simulink model "ARCH_AT6b_artificial"  (R2019b)
settings: Solver=FixedStepAuto  StartTime=0.0  StopTime=10.0  FixedStep=fixedStepSize  RelTol=1e-3
undefined symbols (not defined in the file): ARCH_AT6b_rpmEndTime, ARCH_AT6b_rpmStartTime, ARCH_AT6b_rpmThreshold, ARCH_AT6b_speedEndTime, ARCH_AT6b_speedStartTime, ARCH_AT6b_speedThreshold, artificial_ARCH_AT6_constant
settings Model: Creator=JEDDELAN  LastModifiedBy=JEDDELAN
settings DataIOCC: SaveOutput=off  SaveTime=off  ReturnWorkspaceOutputs=off
settings DebuggingCC: ArithmeticOperatorsInVariantConditions=warning
settings SFSimCC: SimUseLocalCustomCode=off  CustomCodeUndefinedFunction=UseInterfaceOnly
settings RTWCC: RTWUseLocalCustomCode=off
settings GRTTargetCC: CombineOutputUpdateFcns=off  MatFileLogging=off

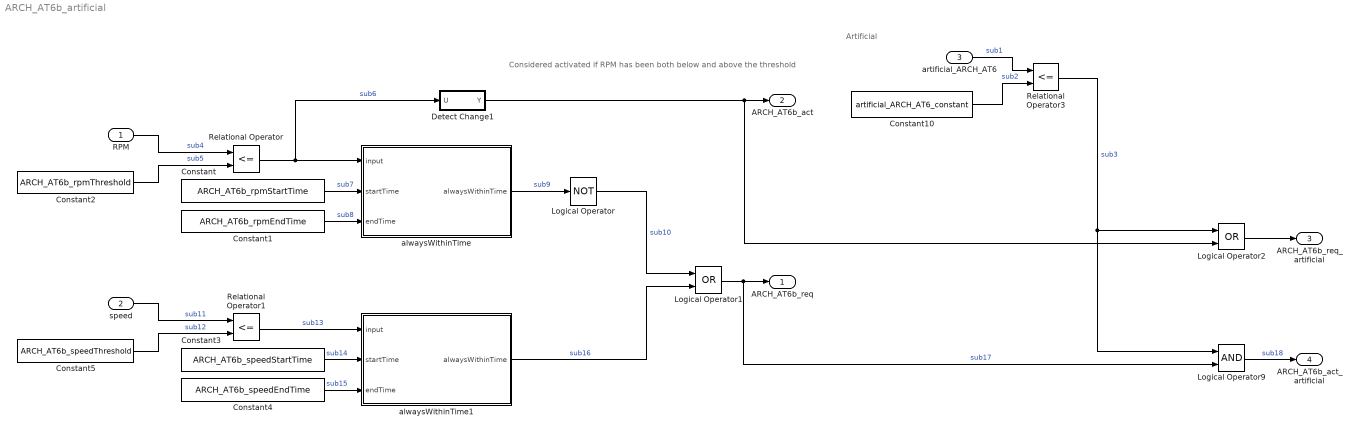
== system ARCH_AT6b_artificial ==
  note: Considered activated if RPM has been both below and above the threshold
  note: Artificial
  RPM : Inport
  speed : Inport  Port=2
  artificial_ARCH_AT6 : Inport  Port=3
  Constant : Constant  Value=ARCH_AT6b_rpmStartTime
  Constant1 : Constant  Value=ARCH_AT6b_rpmEndTime
  Constant10 : Constant  Value=artificial_ARCH_AT6_constant
  Constant2 : Constant  Value=ARCH_AT6b_rpmThreshold
  Constant3 : Constant  Value=ARCH_AT6b_speedStartTime
  Constant4 : Constant  Value=ARCH_AT6b_speedEndTime
  Constant5 : Constant  Value=ARCH_AT6b_speedThreshold
  Detect Change1 : Subsystem  mask(Detect Change){vinit=0, InputProcessing=Elements as channels (sample based), OutDataTypeStr=boolean}
      mask prompts: vinit "Simulink:masks:InitialCondition_MP"; InputProcessing "Simulink:masks:InputProcessing_MP"; OutDataTypeStr "Simulink:masks:OutputDataType_MP"
      mask help: Simulink:masks:DetectChange_MD
      mask init:
      | initDetectBlocks();
      mask TypeOptions InputProcessing: Simulink:masks:ColumnsAsChannelsFrameBased | Simulink:masks:ElementsAsChannelsSampleBased
      mask TypeOptions OutDataTypeStr: Simulink:masks:uint8 | Simulink:masks:boolean
      mask Display: fprintf('U ~= U/z')
  Logical Operator : Logic  Operator=NOT  AllPortsSameDT=off  OutDataTypeStr=boolean
  Logical Operator1 : Logic  Operator=OR  AllPortsSameDT=off  OutDataTypeStr=boolean
  Logical Operator2 : Logic  Operator=OR  AllPortsSameDT=off  OutDataTypeStr=boolean
  Logical Operator9 : Logic  AllPortsSameDT=off  OutDataTypeStr=boolean
  Relational Operator : RelationalOperator  Operator=<=  OutDataTypeStr=boolean  RndMeth=Simplest
  Relational Operator1 : RelationalOperator  Operator=<=  OutDataTypeStr=boolean  RndMeth=Simplest
  Relational Operator3 : RelationalOperator  Operator=<=  OutDataTypeStr=boolean  RndMeth=Simplest
  alwaysWithinTime : Subsystem
      settings: CopyFcn=set_param(gcbh,'LinkStatus','none');
  alwaysWithinTime1 : Subsystem
      settings: CopyFcn=set_param(gcbh,'LinkStatus','none');
  ARCH_AT6b_req : Outport  OutDataTypeStr=boolean  PortDimensions=1  VectorParamsAs1DForOutWhenUnconnected=off
  ARCH_AT6b_act : Outport  Port=2  OutDataTypeStr=boolean  PortDimensions=1  VectorParamsAs1DForOutWhenUnconnected=off
  ARCH_AT6b_req_artificial : Outport  Port=3  OutDataTypeStr=boolean  PortDimensions=1  VectorParamsAs1DForOutWhenUnconnected=off
  ARCH_AT6b_act_artificial : Outport  Port=4  OutDataTypeStr=boolean  PortDimensions=1  VectorParamsAs1DForOutWhenUnconnected=off
  wires:
  Constant1/1 -> alwaysWithinTime/3(endTime)  "sub8"
  Constant/1 -> alwaysWithinTime/2(startTime)  "sub7"
  Relational Operator/1 -> Detect Change1/1(U), alwaysWithinTime/1(input)  "sub6"
  alwaysWithinTime/1(alwaysWithinTime) -> Logical Operator/1  "sub9"
  RPM/1 -> Relational Operator/1  "sub4"
  Constant2/1 -> Relational Operator/2  "sub5"
  speed/1 -> Relational Operator1/1  "sub11"
  Relational Operator1/1 -> alwaysWithinTime1/1(input)  "sub13"
  alwaysWithinTime1/1(alwaysWithinTime) -> Logical Operator1/2  "sub16"
  Constant4/1 -> alwaysWithinTime1/3(endTime)  "sub15"
  Constant3/1 -> alwaysWithinTime1/2(startTime)  "sub14"
  Constant5/1 -> Relational Operator1/2  "sub12"
  Logical Operator/1 -> Logical Operator1/1  "sub10"
  Constant10/1 -> Relational Operator3/2  "sub2"
  artificial_ARCH_AT6/1 -> Relational Operator3/1  "sub1"
  Detect Change1/1(Y) -> Logical Operator2/2, ARCH_AT6b_act/1
  Logical Operator9/1 -> ARCH_AT6b_act_artificial/1  "sub18"
  Logical Operator2/1 -> ARCH_AT6b_req_artificial/1
  Logical Operator1/1 -> Logical Operator9/2, ARCH_AT6b_req/1  "sub17"
  Relational Operator3/1 -> Logical Operator9/1, Logical Operator2/1  "sub3"

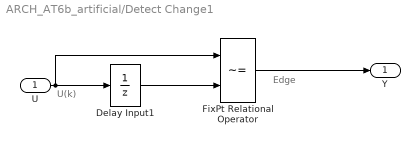
== system ARCH_AT6b_artificial/Detect Change1 ==
  note: Edge
  note: U(k)
  U : Inport
  Delay Input1 : UnitDelay  Description=Store in Global RAM  DisableCoverage=on  InitialCondition=vinit  SampleTime=-1  HasFrameUpgradeWarning=on
  FixPt Relational Operator : RelationalOperator  Operator=~=  OutDataTypeStr=boolean  ZeroCross=off  RndMeth=Nearest
  Y : Outport  InitialOutput=0
  wires:
  FixPt Relational Operator/1 -> Y/1
  Delay Input1/1 -> FixPt Relational Operator/2
  U/1 -> FixPt Relational Operator/1, Delay Input1/1

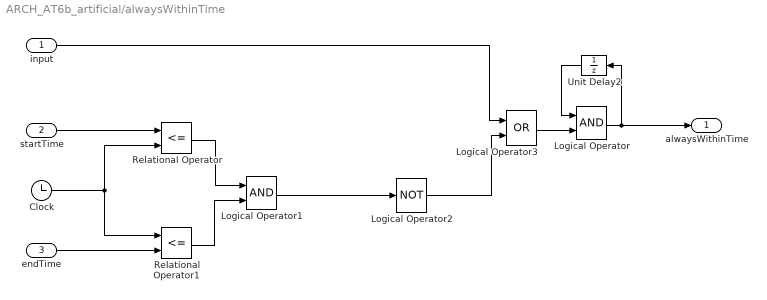
== system ARCH_AT6b_artificial/alwaysWithinTime ==
  input : Inport
  startTime : Inport  Port=2
  endTime : Inport  Port=3
  Clock : Clock
  Logical Operator : Logic  AllPortsSameDT=off  OutDataTypeStr=boolean
  Logical Operator1 : Logic  AllPortsSameDT=off  OutDataTypeStr=boolean
  Logical Operator2 : Logic  Operator=NOT  AllPortsSameDT=off  OutDataTypeStr=boolean
  Logical Operator3 : Logic  Operator=OR  AllPortsSameDT=off  OutDataTypeStr=boolean
  Relational Operator : RelationalOperator  Operator=<=  OutDataTypeStr=boolean  RndMeth=Simplest
  Relational Operator1 : RelationalOperator  Operator=<=  OutDataTypeStr=boolean  RndMeth=Simplest
  Unit Delay2 : UnitDelay  InitialCondition=1  SampleTime=-1  HasFrameUpgradeWarning=on
  alwaysWithinTime : Outport  VectorParamsAs1DForOutWhenUnconnected=off
  wires:
  startTime/1 -> Relational Operator/1
  Clock/1 -> Relational Operator1/1, Relational Operator/2
  endTime/1 -> Relational Operator1/2
  Relational Operator1/1 -> Logical Operator1/2
  Relational Operator/1 -> Logical Operator1/1
  Logical Operator1/1 -> Logical Operator2/1
  Logical Operator2/1 -> Logical Operator3/2
  Logical Operator3/1 -> Logical Operator/2
  Logical Operator/1 -> alwaysWithinTime/1, Unit Delay2/1
  Unit Delay2/1 -> Logical Operator/1
  input/1 -> Logical Operator3/1

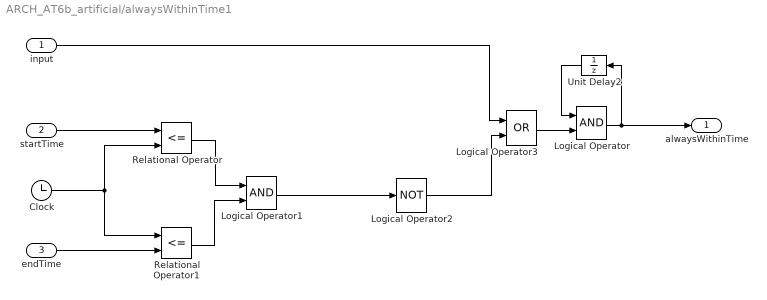
== system ARCH_AT6b_artificial/alwaysWithinTime1 ==
  input : Inport
  startTime : Inport  Port=2
  endTime : Inport  Port=3
  Clock : Clock
  Logical Operator : Logic  AllPortsSameDT=off  OutDataTypeStr=boolean
  Logical Operator1 : Logic  AllPortsSameDT=off  OutDataTypeStr=boolean
  Logical Operator2 : Logic  Operator=NOT  AllPortsSameDT=off  OutDataTypeStr=boolean
  Logical Operator3 : Logic  Operator=OR  AllPortsSameDT=off  OutDataTypeStr=boolean
  Relational Operator : RelationalOperator  Operator=<=  OutDataTypeStr=boolean  RndMeth=Simplest
  Relational Operator1 : RelationalOperator  Operator=<=  OutDataTypeStr=boolean  RndMeth=Simplest
  Unit Delay2 : UnitDelay  InitialCondition=1  SampleTime=-1  HasFrameUpgradeWarning=on
  alwaysWithinTime : Outport  VectorParamsAs1DForOutWhenUnconnected=off
  wires:
  startTime/1 -> Relational Operator/1
  Clock/1 -> Relational Operator1/1, Relational Operator/2
  endTime/1 -> Relational Operator1/2
  Relational Operator1/1 -> Logical Operator1/2
  Relational Operator/1 -> Logical Operator1/1
  Logical Operator1/1 -> Logical Operator2/1
  Logical Operator2/1 -> Logical Operator3/2
  Logical Operator3/1 -> Logical Operator/2
  Logical Operator/1 -> alwaysWithinTime/1, Unit Delay2/1
  Unit Delay2/1 -> Logical Operator/1
  input/1 -> Logical Operator3/1
